simulink model "mbd_example_timer"  (R2022b)
settings: Solver=FixedStepDiscrete  StartTime=0.0  StopTime=10.0  RelTol=1e-3  EnableMultiTasking=on
PostLoadFcn:
  | run([bdroot '_init']);
InitFcn:
  | checkModelFolder(true); % Optional
  | run([bdroot '_init']);
values from neighbouring files (symbols this model uses):
  MBDDiag_Comm_Module = [2 3]    [mbd_example_timer_init.m]
  MBDDiag_Comm_Speed = [921600 921600]    [mbd_example_timer_init.m]
  MBDDiag_Comm_Type = [1 1]    [mbd_example_timer_init.m]
  T_s_LED1 = 1/LED1_Hz    (= 0.5)    [mbd_example_timer_init.m]
  T_s_LED2 = 1/LED2_Hz    (= 1)    [mbd_example_timer_init.m]
libraries: MbdLib_Uart x10, MbdLib_Timer x8, MbdLib_Digital x6, MbdLib_PortalDiag x4, MbdLib_SnapDiag x2, MbdLib_Required x1
settings Model: Creator=KenYoshioka  LastModifiedBy=KenYoshioka
settings SolverCC: AutoInsertRateTranBlk=on
settings OptimizationCC: DefaultParameterBehavior=Inlined  DefaultUnderspecifiedDataType=single  EnhancedBackFolding=on  BooleansAsBitfields=on  PassReuseOutputArgsAs=Individual arguments  ZeroExternalMemoryAtStartup=off  ZeroInternalMemoryAtStartup=off  OptimizeBlockOrder=speed  DifferentSizesBufferReuse=on  EfficientTunableParamExpr=on
settings DebuggingCC: ParameterTunabilityLossMsg=error
settings HardwareCC: ProdBitPerPointer=32  ProdBitPerSizeT=32  ProdBitPerPtrDiffT=32  ProdLargestAtomicInteger=Long  ProdLargestAtomicFloat=Double  ProdWordSize=32  ProdHWDeviceType=ARM Compatible->ARM Cortex-M
settings ModelReferenceCC: ModelReferenceNumInstancesAllowed=Single
settings SFSimCC: MATLABDynamicMemAlloc=off
settings RTWCC: Description=MBD Embedded Target STM32 Cortex M4 (real-time)  SystemTargetFile=MBD_STM32_stf.tlc  TemplateMakefile=MBD_STM32.tmf  Toolchain=arm-none-eabi - v10.3
settings CodeAppCC: ForceParamTrailComments=on  IgnoreCustomStorageClasses=off  MaxIdLength=255  OperatorAnnotations=on  SimulinkDataObjDesc=on  SFDataObjDesc=on  InsertBlockDesc=on
settings STFCustomTargetCC: MultiwordLength=256  IncludeMdlTerminateFcn=off  CombineOutputUpdateFcns=on  CombineSignalStateStructs=on  SuppressErrorStatus=on  ERTCustomFileBanners=on  SupportContinuousTime=off  RemoveResetFunc=on  MATLABClassNameForMDSCustomization=Simulink.SoftwareTarget.ERTCustomization  UseToolchainInfoCompliant=on  SystemTargetFile=MBD_STM32_stf.tlc
settings ERTTargetCC: ParMdlRefBuildCompliant=off  CompOptLevelCompliant=off  ConcurrentExecutionCompliant=off  IncludeMdlTerminateFcn=off  CombineSignalStateStructs=on  SuppressErrorStatus=on  SupportNonInlinedSFcns=on  ModelStepFunctionPrototypeControlCompliant=off  CPPClassGenCompliant=off  ExtModeStaticAllocSize=2000  InlinedParameterPlacement=NonHierarchical  ERTCustomFileTemplate=mbd_lib_interface.tlc  MaxLineWidth=110

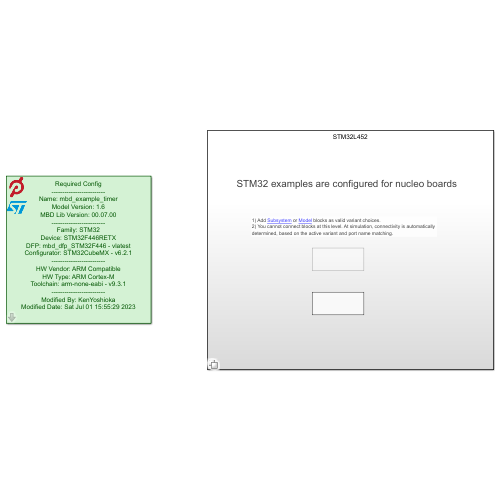
[thumbnail: Simulink's stored preview of the top-level diagram]
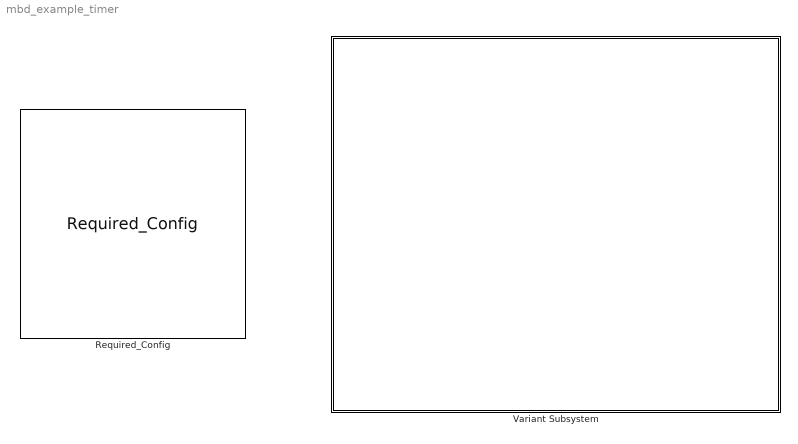
== system mbd_example_timer ==
  Required_Config : MbdLib_Required/Required_Config  Tag=MBD_Target_Info  Param_update=1
      settings: SourceProductName=Peloton Interface Library
  Variant Subsystem : Subsystem  Variant=on

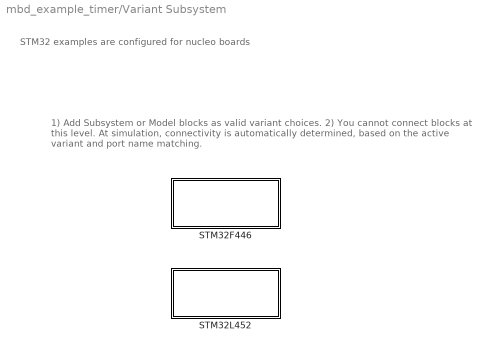
== system mbd_example_timer/Variant Subsystem ==
  note: STM32 examples are configured for nucleo boards
  note: 1) Add Subsystem or Model blocks as valid variant choices.
      | 2) You cannot connect blocks at this level. At simulation, connectivity is automatically
      | determined, based on the active variant and port name matching.
  STM32F446 : Subsystem  VariantControl=VAR_MBD_STM32F446
  STM32L452 : Subsystem  VariantControl=VAR_MBD_STM32L452

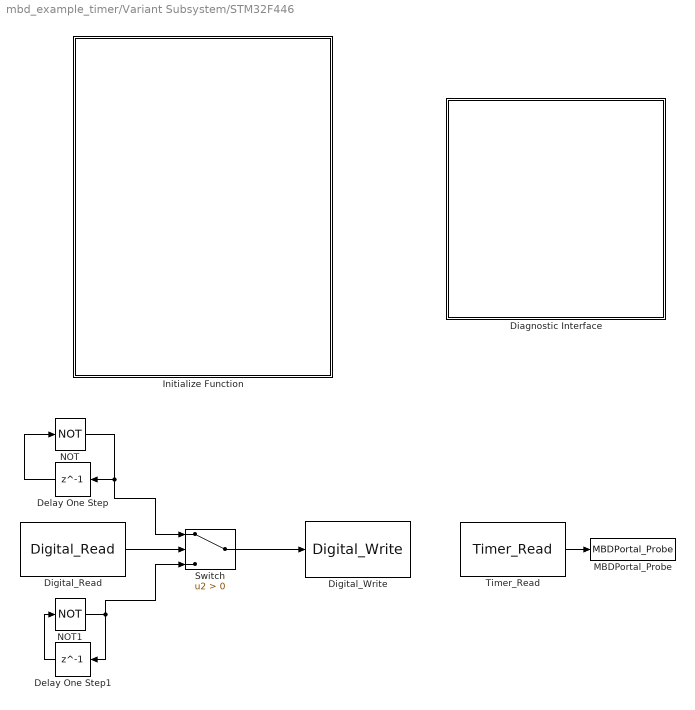
== system mbd_example_timer/Variant Subsystem/STM32F446 ==
  Delay One Step : Delay  DelayLength=1  SampleTime=T_s_LED1
  Delay One Step1 : Delay  DelayLength=1  SampleTime=T_s_LED2
  Diagnostic Interface : Subsystem
  Digital_Read : MbdLib_Digital/Digital_Read  Param_module=C  Param_ch=13  Param_sampleTime=-1  Sim_invert=off  Sim_out=0
      settings: SourceProductName=Peloton Interface Library
  Digital_Write : MbdLib_Digital/Digital_Write  Param_module=C  Param_ch=10  Param_sampleTime=-1
      settings: SourceProductName=Peloton Interface Library
  Initialize Function : Subsystem  TreatAsAtomicUnit=on
  MBDPortal_Probe : MbdLib_PortalDiag/MBDPortal_Probe  Param_SigNameInherited=on  Param_SigName=Timer_out  Param_SigIndex=0  Param_SigMax=MBDPortal_SignalNum  Param_SampleTime=MBDPortal_CommonSampleRate
      settings: SourceProductName=Peloton Component Library
  NOT : Logic  Operator=NOT  IconShape=distinctive  AllPortsSameDT=off  OutDataTypeStr=boolean
  NOT1 : Logic  Operator=NOT  IconShape=distinctive  AllPortsSameDT=off  OutDataTypeStr=boolean
  Switch : Switch  Criteria=u2 > Threshold  SaturateOnIntegerOverflow=off  InputSameDT=off
  Timer_Read : MbdLib_Timer/Timer_Read  Param_module=6  Param_ch=0  Param_sampleTime=-1
      settings: SourceProductName=Peloton Interface Library
  wires:
  NOT1/1 -> Switch/3, Delay One Step1/1
  NOT/1 -> Switch/1, Delay One Step/1
  Delay One Step/1 -> NOT/1
  Delay One Step1/1 -> NOT1/1
  Digital_Read/1 -> Switch/2
  Switch/1 -> Digital_Write/1
  Timer_Read/1 -> MBDPortal_Probe/1

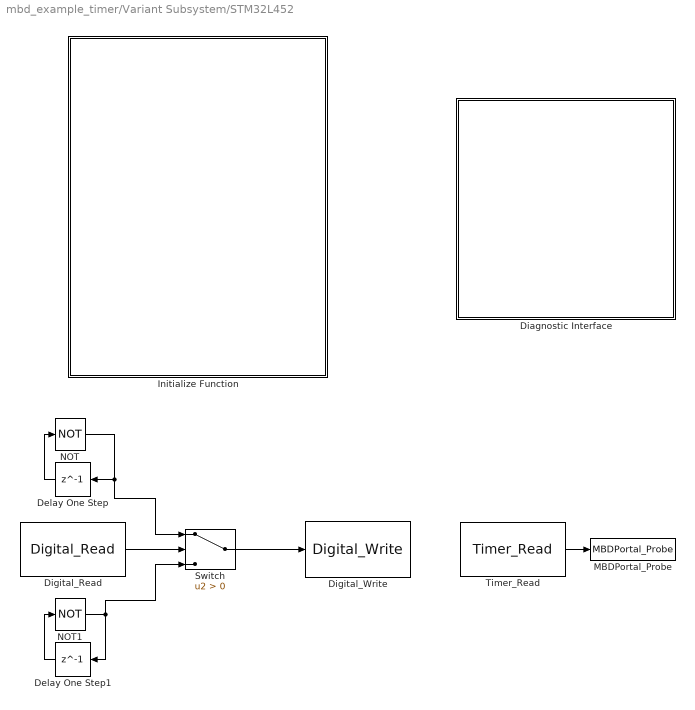
== system mbd_example_timer/Variant Subsystem/STM32L452 ==
  Delay One Step : Delay  DelayLength=1  SampleTime=T_s_LED1
  Delay One Step1 : Delay  DelayLength=1  SampleTime=T_s_LED2
  Diagnostic Interface : Subsystem
  Digital_Read : MbdLib_Digital/Digital_Read  Param_module=C  Param_ch=13  Param_sampleTime=-1  Sim_invert=off  Sim_out=0
      settings: SourceProductName=Peloton Interface Library
  Digital_Write : MbdLib_Digital/Digital_Write  Param_module=C  Param_ch=10  Param_sampleTime=-1
      settings: SourceProductName=Peloton Interface Library
  Initialize Function : Subsystem  TreatAsAtomicUnit=on
  MBDPortal_Probe : MbdLib_PortalDiag/MBDPortal_Probe  Param_SigNameInherited=on  Param_SigName=Timer_out  Param_SigIndex=0  Param_SigMax=MBDPortal_SignalNum  Param_SampleTime=MBDPortal_CommonSampleRate
      settings: SourceProductName=Peloton Component Library
  NOT : Logic  Operator=NOT  IconShape=distinctive  AllPortsSameDT=off  OutDataTypeStr=boolean
  NOT1 : Logic  Operator=NOT  IconShape=distinctive  AllPortsSameDT=off  OutDataTypeStr=boolean
  Switch : Switch  Criteria=u2 > Threshold  SaturateOnIntegerOverflow=off  InputSameDT=off
  Timer_Read : MbdLib_Timer/Timer_Read  Param_module=16  Param_ch=0  Param_sampleTime=-1
      settings: SourceProductName=Peloton Interface Library
  wires:
  NOT1/1 -> Switch/3, Delay One Step1/1
  NOT/1 -> Switch/1, Delay One Step/1
  Delay One Step/1 -> NOT/1
  Delay One Step1/1 -> NOT1/1
  Digital_Read/1 -> Switch/2
  Switch/1 -> Digital_Write/1
  Timer_Read/1 -> MBDPortal_Probe/1

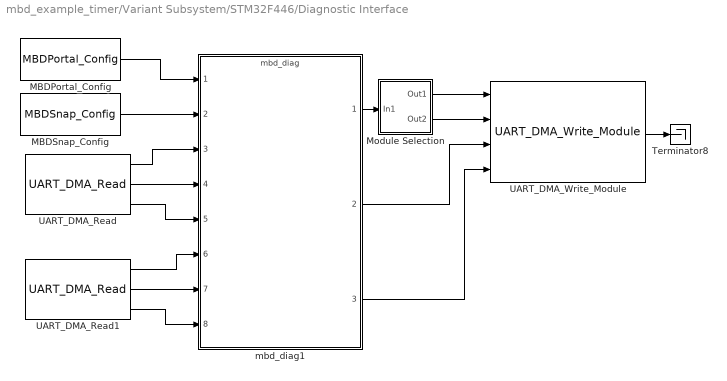
== system mbd_example_timer/Variant Subsystem/STM32F446/Diagnostic Interface ==
  MBDPortal_Config : MbdLib_PortalDiag/MBDPortal_Config  Param_SigMax=MBDPortal_SignalNum  Param_ParamMax=MBDPortal_ParamNum
      settings: SourceProductName=Peloton Component Library
  MBDSnap_Config : MbdLib_SnapDiag/MBDSnap_Config  Priority=-5000  Param_enableAll=on  Param_SampleTime=T_s_COMM  Param_SigMax=MBDSnap_SignalNum
      settings: SourceProductName=Peloton Component Library
  Module Selection : Subsystem
  Terminator8 : Terminator
  UART_DMA_Read : MbdLib_Uart/UART_DMA_Read  Tag=TAG_UART_DMA  Param_module=MBDDiag_Comm_Module(1)  Param_type=USART  Param_readLim=100  Param_sampleTime=T_s_COMM
      settings: SourceProductName=Peloton Interface Library
  UART_DMA_Read1 : MbdLib_Uart/UART_DMA_Read  Tag=TAG_UART_DMA  Param_module=MBDDiag_Comm_Module(2)  Param_type=USART  Param_readLim=100  Param_sampleTime=T_s_COMM
      settings: SourceProductName=Peloton Interface Library
  UART_DMA_Write_Module : MbdLib_Uart/UART_DMA_Write_Module  Param_instanceNum=2  Param_module1=MBDDiag_Comm_Module(1)  Param_type1=USART  Param_module2=MBDDiag_Comm_Module(2)  Param_type2=USART  Param_module3=0  Param_type3=UART  Param_module4=0  Param_type4=UART  Param_sampleTime=-1  Sim_status=0
      settings: SourceProductName=Peloton Interface Library
  mbd_diag1 : ModelReference  ModelNameDialog=mbd_diag.slx  SimulationMode=Normal  ModelReferenceVersion=2.294  SimulationMode=Normal
  wires:
  Module Selection/2(Out2) -> UART_DMA_Write_Module/2
  UART_DMA_Read1/2 -> mbd_diag1/7
  UART_DMA_Read/1 -> mbd_diag1/3
  UART_DMA_Write_Module/1 -> Terminator8/1
  mbd_diag1/1 -> Module Selection/1(In1)
  MBDPortal_Config/1 -> mbd_diag1/1
  mbd_diag1/3 -> UART_DMA_Write_Module/4
  MBDSnap_Config/1 -> mbd_diag1/2
  mbd_diag1/2 -> UART_DMA_Write_Module/3
  UART_DMA_Read/2 -> mbd_diag1/4
  Module Selection/1(Out1) -> UART_DMA_Write_Module/1
  UART_DMA_Read1/1 -> mbd_diag1/6
  UART_DMA_Read/3 -> mbd_diag1/5
  UART_DMA_Read1/3 -> mbd_diag1/8

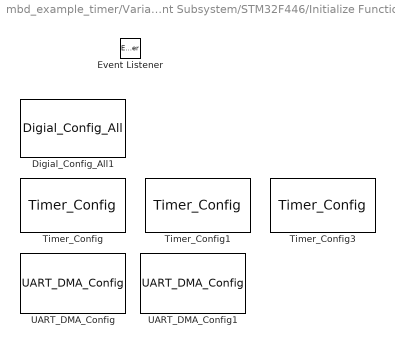
== system mbd_example_timer/Variant Subsystem/STM32F446/Initialize Function ==
  Digial_Config_All1 : MbdLib_Digital/Digial_Config_All  Priority=30  Param_channels={ 'A', '0', 'off', '0 : input', '0 : low', '0 : none', '0 : none', '0 : low', '0 : low'; 'A', '1', 'off', '0 : input', '0 : low', '0 : none', '0 : none', '0 : low', '0 : low'; 'A', '2', 'off', '0 : input', '0 : low', '0 : none', '0 : none', '0 : low', '0 : low'; 'A', '3', 'off', '0 : input', '0 : low', '0 : none', '0 : none', '0 : low', '0 : low'; 'A', '4', 'off', '0 : input', '0 : low', '0 : none', '0 : none', '0 : low', '0 : low'; 'A', '5', 'off', '0 : input', '0 : low', '0 : none', '0 : none', '0 : low', '0 : low'; 'A', '6', 'off', '0 : input', '0 : low', '0 : none', '0 : none', '0 : low', '0 : low'; 'A', '7', 'off', '0 : input', '0 : low', '0 : none', '0 : none', '0 : low', '0 : low'; 'A', '8', 'off', '0 : input', '0 : low', '0 : none', '0 : none', '0 : low', '0 : low'; 'A', '9', 'off', '0 : input', '0 : low', '0 : none', '0 : none', '0 : low', '0 : low'; 'A', '10', 'off', '0 : input', '0 : low', '0 : none', '0 : none', '0 : low', '0 : low'; 'A', '11', 'off', '0 : input', '0 : low', '0 : none', '0 : none', '0 : low', '0 : low'; 'A', '12', 'off', '0 : input', '0 : low', '0 : none', '0 : none', '0 : low', '0 : low'; 'A', '13', 'off', '0 : input', '0 : low', '0 : none', '0 : none', '0 : low', '0 : low'; 'A', '14', 'off', '0 : input', '0 : low', '0 : none', '0 : none', '0 : low', '0 : low'; 'A', '15', 'off', '0 : input', '0 : low', '0 : none', '0 : none', '0 : low', '0 : low'; 'A', '16', 'off', '0 : input', '0 : low', '0 : none', '0 : none', '0 : low', '0 : low'; 'A', '17', 'off', '0 : input', '0 : low', '0 : none', '0 : none', '0 : low', '0 : low'; 'A', '18', 'off', '0 : input', '0 : low', '0 : none', '0 : none', '0 : low', '0 : low'; 'A', '19', 'off', '0 : input', '0 : low', '0 : none', '0 : none', '0 : low', '0 : low'; 'A', '20', 'off', '0 : input', '0 : low', '0 : none', '0 : none', '0 : low', '0 : low'; 'A', '21', 'off', '0 : input', '0 : low', '0 : none', '0 : none', '0 : low', '0 : low'; 'A', '22', 'off', '0 : input', '0 : low', '0 : none', '0 : none', '0 : low', '0 : low'; 'A', '23', 'off', '0 : input', '0 : low', '0 : none', '0 : none', '0 : low', '0 : low'; 'A', '24', 'off', '0 : input', '0 : low', '0 : none', '0 : none', '0 : low', '0 : low'; 'A', '25', 'off', '0 : input', '0 : low', '0 : none', '0 : none', '0 : low', '0 : low'; 'A', '26', 'off', '0 : input', '0 : low', '0 : none', '0 : none', '0 : low', '0 : low'; 'A', '27', 'off', '0 : input', '0 : low', '0 : none', '0 : none', '0 : low', '0 : low'; 'A', '28', 'off', '0 : input', '0 : low', '0 : none', '0 : none', '0 : low', '0 : low'; 'A', '29', 'off', '0 : input', '0 : low', '0 : none', '0 : none', '0 : low', '0 : low'; 'A', '30', 'off', '0 : input', '0 : low', '0 : none', '0 : none', '0 : low', '0 : low'; 'A', '31', 'off', '0 : input', '0 : low', '0 : none', '0 : none', '0 : low', '0 : low'; 'B', '0', 'off', '0 : input', '0 : low', '0 : none', '0 : none', '0 : low', '0 : low'; 'B', '1', 'off', '0 : input', '0 : low', '0 : none', '0 : none', '0 : low', '0 : low'; 'B', '2', 'off', '0 : input', '0 : low', '0 : none', '0 : none', '0 : low', '0 : low'; 'B', '3', 'off', '0 : input', '0 : low', '0 : none', '0 : none', '0 : low', '0 : low'; 'B', '4', 'off', '0 : input', '0 : low', '0 : none', '0 : none', '0 : low', '0 : low'; 'B', '5', 'off', '0 : input', '0 : low', '0 : none', '0 : none', '0 : low', '0 : low'; 'B', '6', 'off', '0 : input', '0 : low', '0 : none', '0 : none', '0 : low', '0 : low'; 'B', '7', 'off', '0 : input', '0 : low', '0 : none', '0 : none', '0 : low', '0 : low'; 'B', '8', 'off', '0 : input', '0 : low', '0 : none', '0 : none', '0 : low', '0 : low'; 'B', '9', 'off', '0 : input', '0 : low', '0 : none', '0 : none', '0 : low', '0 : low'; 'B', '10', 'off', '0 : input', '0 : low', '0 : none', '0 : none', '0 : low', '0 : low'; 'B', '11', 'off', '0 : input', '0 : low', '0 : none', '0 : none', '0 : low', '0 : low'; 'B', '12', 'off', '0 : input', '0 : low', '0 : none', '0 : none', '0 : low', '0 : low'; 'B', '13', 'off', '0 : input', '0 : low', '0 : none', '0 : none', '0 : low', '0 : low'; 'C', '0', 'off', '0 : input', '0 : low', '0 : none', '0 : none', '0 : low', '0 : low'; 'C', '1', 'off', '0 : input', '0 : low', '0 : none', '0 : none', '0 : low', '0 : low'; 'C', '2', 'off', '0 : input', '0 : low', '0 : none', '0 : none', '0 : low', '0 : low'; 'C', '3', 'off', '0 : input', '0 : low', '0 : none', '0 : none', '0 : low', '0 : low'; 'C', '4', 'off', '0 : input', '0 : low', '0 : none', '0 : none', '0 : low', '0 : low'; 'C', '5', 'off', '0 : input', '0 : low', '0 : none', '0 : none', '0 : low', '0 : low'; 'C', '6', 'off', '0 : input', '0 : low', '0 : none', '0 : none', '0 : low', '0 : low'; 'C', '7', 'off', '0 : input', '0 : low', '0 : none', '0 : none', '0 : low', '0 : low'; 'C', '8', 'off', '0 : input', '0 : low', '0 : none', '0 : none', '0 : low', '0 : low'; 'C', '9', 'off', '0 : input', '0 : low', '0 : none', '0 : none', '0 : low', '0 : low'; 'C', '10', 'on', '1 : output', '0 : low', '0 : none', '0 : none', '0 : low', '0 : low'; 'C', '11', 'off', '0 : input', '0 : low', '0 : none', '0 : none', '0 : low', '0 : low'; 'C', '12', 'off', '0 : input', '0 : low', '0 : none', '0 : none', '0 : low', '0 : low'; 'C', '13', 'on', '0 : input', '0 : low', '0 : none', '1 : pullup', '0 : low', '0 : low'; 'C', '14', 'off', '0 : input', '0 : low', '0 : none', '0 : none', '0 : low', '0 : low'; 'C', '15', 'off', '0 : input', '0 : low', '0 : none', '0 : none', '0 : low', '0 : low'; 'C', '16', 'off', '0 : input', '0 : low', '0 : none', '0 : none', '0 : low', '0 : low'; 'C', '17', 'off', '0 : input', '0 : low', '0 : none', '0 : none', '0 : low', '0 : low'; 'C', '18', 'off', '0 : input', '0 : low', '0 : none', '0 : none', '0 : low', '0 : low'; 'C', '19', 'off', '0 : input', '0 : low', '0 : none', '0 : none', '0 : low', '0 : low'; 'C', '20', 'off', '0 : input', '0 : low', '0 : none', '0 : none', '0 : low', '0 : low'; 'C', '21', 'off', '0 : input', '0 : low', '0 : none', '0 : none', '0 : low', '0 : low'; 'C', '22', 'off', '0 : input', '0 : low', '0 : none', '0 : none', '0 : low', '0 : low'; 'C', '23', 'off', '0 : input', '0 : low', '0 : none', '0 : none', '0 : low', '0 : low'; 'C', '24', 'off', '0 : input', '0 : low', '0 : none', '0 : none', '0 : low', '0 : low'; 'C', '25', 'off', '0 : input', '0 : low', '0 : none', '0 : none', '0 : low', '0 : low'; 'C', '26', 'off', '0 : input', '0 : low', '0 : none', '0 : none', '0 : low', '0 : low'; 'C', '27', 'off', '0 : input', '0 : low', '0 : none', '0 : none', '0 : low', '0 : low'; 'C', '28', 'off', '0 : input', '0 : low', '0 : none', '0 : none', '0 : low', '0 : low'; 'C', '29', 'off', '0 : input', '0 : low', '0 : none', '0 : none', '0 : low', '0 : low'; 'C', '30', 'off', '0 : input', '0 : low', '0 : none', '0 : none', '0 : low', '0 : low'; 'C', '31', 'off', '0 : input', '0 : low', '0 : none', '0 : none', '0 : low', '0 : low'; 'D', '0', 'off', '0 : input', '0 : low', '0 : none', '0 : none', '0 : low', '0 : low'; 'D', '1', 'off', '0 : input', '0 : low', '0 : none', '0 : none', '0 : low', '0 : low'; 'D', '2', 'off', '0 : input', '0 : low', '0 : none', '0 : none', '0 : low', '0 : low'; 'D', '3', 'off', '0 : input', '0 : low', '0 : none', '0 : none', '0 : low', '0 : low'; 'D', '4', 'off', '0 : input', '0 : low', '0 : none', '0 : none', '0 : low', '0 : low'; 'D', '5', 'off', '0 : input', '0 : low', '0 : none', '0 : none', '0 : low', '0 : low'; 'D', '6', 'off', '0 : input', '0 : low', '0 : none', '0 : none', '0 : low', '0 : low'; 'D', '7', 'off', '0 : input', '0 : low', '0 : none', '0 : none', '0 : low', '0 : low'; 'D', '8', 'off', '0 : input', '0 : low', '0 : none', '0 : none', '0 : low', '0 : low'; 'D', '9', 'off', '0 : input', '0 : low', '0 : none', '0 : none', '0 : low', '0 : low'; 'D', '10', 'off', '0 : input', '0 : low', '0 : none', '0 : none', '0 : low', '0 : low'; 'D', '11', 'off', '0 : input', '0 : low', '0 : none', '0 : none', '0 : low', '0 : low'; 'D', '12', 'off', '0 : input', '0 : low', '0 : none', '0 : none', '0 : low', '0 : low'; 'D', '13', 'off', '0 : input', '0 : low', '0 : none', '0 : none', '0 : low', '0 : low'; 'D', '14', 'off', '0 : input', '0 : low', '0 : none', '0 : none', '0 : low', '0 : low'; 'D', '15', 'off', '0 : input', '0 : low', '0 : none', '0 : none', '0 : low', '0 : low'; 'D', '16', 'off', '0 : input', '0 : low', '0 : none', '0 : none', '0 : low', '0 : low'; 'D', '17', 'off', '0 : input', '0 : low', '0 : none', '0 : none', '0 : low', '0 : low'; 'D', '18', 'off', '0 : input', '0 : low', '0 : none', '0 : none', '0 : low', '0 : low'; 'D', '19', 'off', '0 : input', '0 : low', '0 : none', '0 : none', '0 : low', '0 : low'; 'D', '20', 'off', '0 : input', '0 : low', '0 : none', '0 : none', '0 : low', '0 : low'; 'D', '21', 'off', '0 : input', '0 : low', '0 : none', '0 : none', '0 : low', '0 : low'; 'D', '22', 'off', '0 : input', '0 : low', '0 : none', '0 : none', '0 : low', '0 : low'; 'D', '23', 'off', '0 : input', '0 : low', '0 : none', '0 : none', '0 : low', '0 : low'; 'D', '24', 'off', '0 : input', '0 : low', '0 : none', '0 : none', '0 : low', '0 : low'; 'D', '25', 'off', '0 : input', '0 : low', '0 : none', '0 : none', '0 : low', '0 : low'; 'D', '26', 'off', '0 : input', '0 : low', '0 : none', '0 : none', '0 : low', '0 : low'; 'D', '27', 'off', '0 : input', '0 : low', '0 : none', '0 : none', '0 : low', '0 : low'; 'D', '28', 'off', '0 : input', '0 : low', '0 : none', '0 : none', '0 : low', '0 : low'; 'D', '29', 'off', '0 : input', '0 : low', '0 : none', '0 : none', '0 : low', '0 : low'; 'D', '30', 'off', '0 : input', '0 : low', '0 : none', '0 : none', '0 : low', '0 : low'; 'D', '31', 'off', '0 : input', '0 : low', '0 : none', '0 : none', '0 : low', '0 : low'; 'E', '0', 'off', '0 : input', '0 : low', '0 : none', '0 : none', '0 : low', '0 : low'; 'E', '1', 'off', '0 : input', '0 : low', '0 : none', '0 : none', '0 : low', '0 : low'; 'E', '2', 'off', '0 : input', '0 : low', '0 : none', '0 : none', '0 : low', '0 : low'; 'E', '3', 'off', '0 : input', '0 : low', '0 : none', '0 : none', '0 : low', '0 : low'; 'E', '4', 'off', '0 : input', '0 : low', '0 : none', '0 : none', '0 : low', '0 : low'; 'E', '5', 'off', '0 : input', '0 : low', '0 : none', '0 : none', '0 : low', '0 : low' }  Param_priority=30  Param_sampleTime=-1
      settings: AttributesFormatString=priority=%<priority>  SourceProductName=Peloton Interface Library
  Event Listener : EventListener  DisableCoverage=on  EventName=reset
  Timer_Config : MbdLib_Timer/Timer_Config  Priority=100  Param_update=1  Param_module=1  Param_step=0  Param_period=Comm_period_cycles  Param_divider=Comm_clock_divider  Param_step0=0  Param_clksrc0=0  Param_period0=LED1_period_cycles  Param_divider0=LED1_clock_divider  Param_step1=-1  Param_clksrc1=0  Param_period1=0  Param_divider1=0  Param_step2=-1  Param_clksrc2=0  Param_period2=0  Param_divider2=0  Param_priority=100  Param_sampleTime=-1
      settings: AttributesFormatString=priority=%<priority>  SourceProductName=Peloton Interface Library
  Timer_Config1 : MbdLib_Timer/Timer_Config  Priority=101  Param_update=1  Param_module=6  Param_step=1  Param_period=LED1_period_cycles  Param_divider=LED1_clock_divider  Param_step0=1  Param_clksrc0=0  Param_period0=LED2_period_cycles  Param_divider0=LED2_clock_divider  Param_step1=-1  Param_clksrc1=0  Param_period1=0  Param_divider1=0  Param_step2=-1  Param_clksrc2=0  Param_period2=0  Param_divider2=0  Param_priority=101  Param_sampleTime=-1
      settings: AttributesFormatString=priority=%<priority>  SourceProductName=Peloton Interface Library
  Timer_Config3 : MbdLib_Timer/Timer_Config  Priority=102  Param_update=1  Param_module=7  Param_step=2  Param_period=LED2_period_cycles  Param_divider=LED2_clock_divider  Param_step0=2  Param_clksrc0=0  Param_period0=LED2_period_cycles  Param_divider0=LED2_clock_divider  Param_step1=-1  Param_clksrc1=0  Param_period1=0  Param_divider1=0  Param_step2=-1  Param_clksrc2=0  Param_period2=0  Param_divider2=0  Param_priority=102  Param_sampleTime=-1
      settings: AttributesFormatString=priority=%<priority>  SourceProductName=Peloton Interface Library
  UART_DMA_Config : MbdLib_Uart/UART_DMA_Config  Priority=110  Param_module=MBDDiag_Comm_Module(1)  Param_type=USART  Param_speed=MBDDiag_Comm_Speed(1)  Param_dataBits=8  Param_stopBits=1  Param_parity=None  Param_priority=110  Param_sampleTime=-1
      settings: AttributesFormatString=priority=%<priority>  SourceProductName=Peloton Interface Library
  UART_DMA_Config1 : MbdLib_Uart/UART_DMA_Config  Priority=110  Param_module=MBDDiag_Comm_Module(2)  Param_type=USART  Param_speed=MBDDiag_Comm_Speed(2)  Param_dataBits=8  Param_stopBits=1  Param_parity=None  Param_priority=110  Param_sampleTime=-1
      settings: AttributesFormatString=priority=%<priority>  SourceProductName=Peloton Interface Library

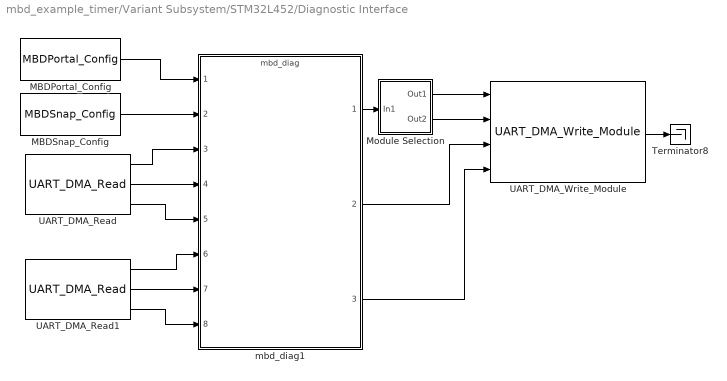
== system mbd_example_timer/Variant Subsystem/STM32L452/Diagnostic Interface ==
  MBDPortal_Config : MbdLib_PortalDiag/MBDPortal_Config  Param_SigMax=MBDPortal_SignalNum  Param_ParamMax=MBDPortal_ParamNum
      settings: SourceProductName=Peloton Component Library
  MBDSnap_Config : MbdLib_SnapDiag/MBDSnap_Config  Priority=-5000  Param_enableAll=on  Param_SampleTime=T_s_COMM  Param_SigMax=MBDSnap_SignalNum
      settings: SourceProductName=Peloton Component Library
  Module Selection : Subsystem
  Terminator8 : Terminator
  UART_DMA_Read : MbdLib_Uart/UART_DMA_Read  Tag=TAG_UART_DMA  Param_module=MBDDiag_Comm_Module(1)  Param_type=USART  Param_readLim=100  Param_sampleTime=T_s_COMM
      settings: SourceProductName=Peloton Interface Library
  UART_DMA_Read1 : MbdLib_Uart/UART_DMA_Read  Tag=TAG_UART_DMA  Param_module=MBDDiag_Comm_Module(2)  Param_type=USART  Param_readLim=100  Param_sampleTime=T_s_COMM
      settings: SourceProductName=Peloton Interface Library
  UART_DMA_Write_Module : MbdLib_Uart/UART_DMA_Write_Module  Param_instanceNum=2  Param_module1=MBDDiag_Comm_Module(1)  Param_type1=USART  Param_module2=MBDDiag_Comm_Module(2)  Param_type2=USART  Param_module3=0  Param_type3=UART  Param_module4=0  Param_type4=UART  Param_sampleTime=-1  Sim_status=0
      settings: SourceProductName=Peloton Interface Library
  mbd_diag1 : ModelReference  ModelNameDialog=mbd_diag.slx  SimulationMode=Normal  ModelReferenceVersion=2.294  SimulationMode=Normal
  wires:
  Module Selection/2(Out2) -> UART_DMA_Write_Module/2
  UART_DMA_Read1/2 -> mbd_diag1/7
  UART_DMA_Read/1 -> mbd_diag1/3
  UART_DMA_Write_Module/1 -> Terminator8/1
  mbd_diag1/1 -> Module Selection/1(In1)
  MBDPortal_Config/1 -> mbd_diag1/1
  mbd_diag1/3 -> UART_DMA_Write_Module/4
  MBDSnap_Config/1 -> mbd_diag1/2
  mbd_diag1/2 -> UART_DMA_Write_Module/3
  UART_DMA_Read/2 -> mbd_diag1/4
  Module Selection/1(Out1) -> UART_DMA_Write_Module/1
  UART_DMA_Read1/1 -> mbd_diag1/6
  UART_DMA_Read/3 -> mbd_diag1/5
  UART_DMA_Read1/3 -> mbd_diag1/8

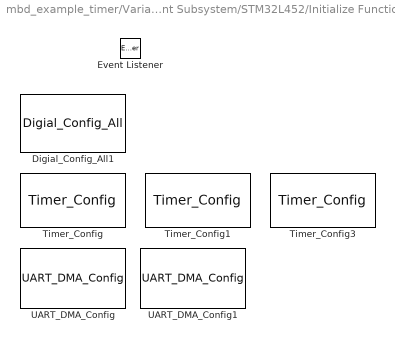
== system mbd_example_timer/Variant Subsystem/STM32L452/Initialize Function ==
  Digial_Config_All1 : MbdLib_Digital/Digial_Config_All  Priority=30  Param_channels={ 'A', '0', 'off', '0 : input', '0 : low', '0 : none', '0 : none', '0 : low', '0 : low'; 'A', '1', 'off', '0 : input', '0 : low', '0 : none', '0 : none', '0 : low', '0 : low'; 'A', '2', 'off', '0 : input', '0 : low', '0 : none', '0 : none', '0 : low', '0 : low'; 'A', '3', 'off', '0 : input', '0 : low', '0 : none', '0 : none', '0 : low', '0 : low'; 'A', '4', 'off', '0 : input', '0 : low', '0 : none', '0 : none', '0 : low', '0 : low'; 'A', '5', 'off', '0 : input', '0 : low', '0 : none', '0 : none', '0 : low', '0 : low'; 'A', '6', 'off', '0 : input', '0 : low', '0 : none', '0 : none', '0 : low', '0 : low'; 'A', '7', 'off', '0 : input', '0 : low', '0 : none', '0 : none', '0 : low', '0 : low'; 'A', '8', 'off', '0 : input', '0 : low', '0 : none', '0 : none', '0 : low', '0 : low'; 'A', '9', 'off', '0 : input', '0 : low', '0 : none', '0 : none', '0 : low', '0 : low'; 'A', '10', 'off', '0 : input', '0 : low', '0 : none', '0 : none', '0 : low', '0 : low'; 'A', '11', 'off', '0 : input', '0 : low', '0 : none', '0 : none', '0 : low', '0 : low'; 'A', '12', 'off', '0 : input', '0 : low', '0 : none', '0 : none', '0 : low', '0 : low'; 'A', '13', 'off', '0 : input', '0 : low', '0 : none', '0 : none', '0 : low', '0 : low'; 'A', '14', 'off', '0 : input', '0 : low', '0 : none', '0 : none', '0 : low', '0 : low'; 'A', '15', 'off', '0 : input', '0 : low', '0 : none', '0 : none', '0 : low', '0 : low'; 'A', '16', 'off', '0 : input', '0 : low', '0 : none', '0 : none', '0 : low', '0 : low'; 'A', '17', 'off', '0 : input', '0 : low', '0 : none', '0 : none', '0 : low', '0 : low'; 'A', '18', 'off', '0 : input', '0 : low', '0 : none', '0 : none', '0 : low', '0 : low'; 'A', '19', 'off', '0 : input', '0 : low', '0 : none', '0 : none', '0 : low', '0 : low'; 'A', '20', 'off', '0 : input', '0 : low', '0 : none', '0 : none', '0 : low', '0 : low'; 'A', '21', 'off', '0 : input', '0 : low', '0 : none', '0 : none', '0 : low', '0 : low'; 'A', '22', 'off', '0 : input', '0 : low', '0 : none', '0 : none', '0 : low', '0 : low'; 'A', '23', 'off', '0 : input', '0 : low', '0 : none', '0 : none', '0 : low', '0 : low'; 'A', '24', 'off', '0 : input', '0 : low', '0 : none', '0 : none', '0 : low', '0 : low'; 'A', '25', 'off', '0 : input', '0 : low', '0 : none', '0 : none', '0 : low', '0 : low'; 'A', '26', 'off', '0 : input', '0 : low', '0 : none', '0 : none', '0 : low', '0 : low'; 'A', '27', 'off', '0 : input', '0 : low', '0 : none', '0 : none', '0 : low', '0 : low'; 'A', '28', 'off', '0 : input', '0 : low', '0 : none', '0 : none', '0 : low', '0 : low'; 'A', '29', 'off', '0 : input', '0 : low', '0 : none', '0 : none', '0 : low', '0 : low'; 'A', '30', 'off', '0 : input', '0 : low', '0 : none', '0 : none', '0 : low', '0 : low'; 'A', '31', 'off', '0 : input', '0 : low', '0 : none', '0 : none', '0 : low', '0 : low'; 'B', '0', 'off', '0 : input', '0 : low', '0 : none', '0 : none', '0 : low', '0 : low'; 'B', '1', 'off', '0 : input', '0 : low', '0 : none', '0 : none', '0 : low', '0 : low'; 'B', '2', 'off', '0 : input', '0 : low', '0 : none', '0 : none', '0 : low', '0 : low'; 'B', '3', 'off', '0 : input', '0 : low', '0 : none', '0 : none', '0 : low', '0 : low'; 'B', '4', 'off', '0 : input', '0 : low', '0 : none', '0 : none', '0 : low', '0 : low'; 'B', '5', 'off', '0 : input', '0 : low', '0 : none', '0 : none', '0 : low', '0 : low'; 'B', '6', 'off', '0 : input', '0 : low', '0 : none', '0 : none', '0 : low', '0 : low'; 'B', '7', 'off', '0 : input', '0 : low', '0 : none', '0 : none', '0 : low', '0 : low'; 'B', '8', 'off', '0 : input', '0 : low', '0 : none', '0 : none', '0 : low', '0 : low'; 'B', '9', 'off', '0 : input', '0 : low', '0 : none', '0 : none', '0 : low', '0 : low'; 'B', '10', 'off', '0 : input', '0 : low', '0 : none', '0 : none', '0 : low', '0 : low'; 'B', '11', 'off', '0 : input', '0 : low', '0 : none', '0 : none', '0 : low', '0 : low'; 'B', '12', 'off', '0 : input', '0 : low', '0 : none', '0 : none', '0 : low', '0 : low'; 'B', '13', 'off', '0 : input', '0 : low', '0 : none', '0 : none', '0 : low', '0 : low'; 'C', '0', 'off', '0 : input', '0 : low', '0 : none', '0 : none', '0 : low', '0 : low'; 'C', '1', 'off', '0 : input', '0 : low', '0 : none', '0 : none', '0 : low', '0 : low'; 'C', '2', 'off', '0 : input', '0 : low', '0 : none', '0 : none', '0 : low', '0 : low'; 'C', '3', 'off', '0 : input', '0 : low', '0 : none', '0 : none', '0 : low', '0 : low'; 'C', '4', 'off', '0 : input', '0 : low', '0 : none', '0 : none', '0 : low', '0 : low'; 'C', '5', 'off', '0 : input', '0 : low', '0 : none', '0 : none', '0 : low', '0 : low'; 'C', '6', 'off', '0 : input', '0 : low', '0 : none', '0 : none', '0 : low', '0 : low'; 'C', '7', 'off', '0 : input', '0 : low', '0 : none', '0 : none', '0 : low', '0 : low'; 'C', '8', 'off', '0 : input', '0 : low', '0 : none', '0 : none', '0 : low', '0 : low'; 'C', '9', 'off', '0 : input', '0 : low', '0 : none', '0 : none', '0 : low', '0 : low'; 'C', '10', 'on', '1 : output', '0 : low', '0 : none', '0 : none', '0 : low', '0 : low'; 'C', '11', 'off', '0 : input', '0 : low', '0 : none', '0 : none', '0 : low', '0 : low'; 'C', '12', 'off', '0 : input', '0 : low', '0 : none', '0 : none', '0 : low', '0 : low'; 'C', '13', 'on', '0 : input', '0 : low', '0 : none', '1 : pullup', '0 : low', '0 : low'; 'C', '14', 'off', '0 : input', '0 : low', '0 : none', '0 : none', '0 : low', '0 : low'; 'C', '15', 'off', '0 : input', '0 : low', '0 : none', '0 : none', '0 : low', '0 : low'; 'C', '16', 'off', '0 : input', '0 : low', '0 : none', '0 : none', '0 : low', '0 : low'; 'C', '17', 'off', '0 : input', '0 : low', '0 : none', '0 : none', '0 : low', '0 : low'; 'C', '18', 'off', '0 : input', '0 : low', '0 : none', '0 : none', '0 : low', '0 : low'; 'C', '19', 'off', '0 : input', '0 : low', '0 : none', '0 : none', '0 : low', '0 : low'; 'C', '20', 'off', '0 : input', '0 : low', '0 : none', '0 : none', '0 : low', '0 : low'; 'C', '21', 'off', '0 : input', '0 : low', '0 : none', '0 : none', '0 : low', '0 : low'; 'C', '22', 'off', '0 : input', '0 : low', '0 : none', '0 : none', '0 : low', '0 : low'; 'C', '23', 'off', '0 : input', '0 : low', '0 : none', '0 : none', '0 : low', '0 : low'; 'C', '24', 'off', '0 : input', '0 : low', '0 : none', '0 : none', '0 : low', '0 : low'; 'C', '25', 'off', '0 : input', '0 : low', '0 : none', '0 : none', '0 : low', '0 : low'; 'C', '26', 'off', '0 : input', '0 : low', '0 : none', '0 : none', '0 : low', '0 : low'; 'C', '27', 'off', '0 : input', '0 : low', '0 : none', '0 : none', '0 : low', '0 : low'; 'C', '28', 'off', '0 : input', '0 : low', '0 : none', '0 : none', '0 : low', '0 : low'; 'C', '29', 'off', '0 : input', '0 : low', '0 : none', '0 : none', '0 : low', '0 : low'; 'C', '30', 'off', '0 : input', '0 : low', '0 : none', '0 : none', '0 : low', '0 : low'; 'C', '31', 'off', '0 : input', '0 : low', '0 : none', '0 : none', '0 : low', '0 : low'; 'D', '0', 'off', '0 : input', '0 : low', '0 : none', '0 : none', '0 : low', '0 : low'; 'D', '1', 'off', '0 : input', '0 : low', '0 : none', '0 : none', '0 : low', '0 : low'; 'D', '2', 'off', '0 : input', '0 : low', '0 : none', '0 : none', '0 : low', '0 : low'; 'D', '3', 'off', '0 : input', '0 : low', '0 : none', '0 : none', '0 : low', '0 : low'; 'D', '4', 'off', '0 : input', '0 : low', '0 : none', '0 : none', '0 : low', '0 : low'; 'D', '5', 'off', '0 : input', '0 : low', '0 : none', '0 : none', '0 : low', '0 : low'; 'D', '6', 'off', '0 : input', '0 : low', '0 : none', '0 : none', '0 : low', '0 : low'; 'D', '7', 'off', '0 : input', '0 : low', '0 : none', '0 : none', '0 : low', '0 : low'; 'D', '8', 'off', '0 : input', '0 : low', '0 : none', '0 : none', '0 : low', '0 : low'; 'D', '9', 'off', '0 : input', '0 : low', '0 : none', '0 : none', '0 : low', '0 : low'; 'D', '10', 'off', '0 : input', '0 : low', '0 : none', '0 : none', '0 : low', '0 : low'; 'D', '11', 'off', '0 : input', '0 : low', '0 : none', '0 : none', '0 : low', '0 : low'; 'D', '12', 'off', '0 : input', '0 : low', '0 : none', '0 : none', '0 : low', '0 : low'; 'D', '13', 'off', '0 : input', '0 : low', '0 : none', '0 : none', '0 : low', '0 : low'; 'D', '14', 'off', '0 : input', '0 : low', '0 : none', '0 : none', '0 : low', '0 : low'; 'D', '15', 'off', '0 : input', '0 : low', '0 : none', '0 : none', '0 : low', '0 : low'; 'D', '16', 'off', '0 : input', '0 : low', '0 : none', '0 : none', '0 : low', '0 : low'; 'D', '17', 'off', '0 : input', '0 : low', '0 : none', '0 : none', '0 : low', '0 : low'; 'D', '18', 'off', '0 : input', '0 : low', '0 : none', '0 : none', '0 : low', '0 : low'; 'D', '19', 'off', '0 : input', '0 : low', '0 : none', '0 : none', '0 : low', '0 : low'; 'D', '20', 'off', '0 : input', '0 : low', '0 : none', '0 : none', '0 : low', '0 : low'; 'D', '21', 'off', '0 : input', '0 : low', '0 : none', '0 : none', '0 : low', '0 : low'; 'D', '22', 'off', '0 : input', '0 : low', '0 : none', '0 : none', '0 : low', '0 : low'; 'D', '23', 'off', '0 : input', '0 : low', '0 : none', '0 : none', '0 : low', '0 : low'; 'D', '24', 'off', '0 : input', '0 : low', '0 : none', '0 : none', '0 : low', '0 : low'; 'D', '25', 'off', '0 : input', '0 : low', '0 : none', '0 : none', '0 : low', '0 : low'; 'D', '26', 'off', '0 : input', '0 : low', '0 : none', '0 : none', '0 : low', '0 : low'; 'D', '27', 'off', '0 : input', '0 : low', '0 : none', '0 : none', '0 : low', '0 : low'; 'D', '28', 'off', '0 : input', '0 : low', '0 : none', '0 : none', '0 : low', '0 : low'; 'D', '29', 'off', '0 : input', '0 : low', '0 : none', '0 : none', '0 : low', '0 : low'; 'D', '30', 'off', '0 : input', '0 : low', '0 : none', '0 : none', '0 : low', '0 : low'; 'D', '31', 'off', '0 : input', '0 : low', '0 : none', '0 : none', '0 : low', '0 : low'; 'E', '0', 'off', '0 : input', '0 : low', '0 : none', '0 : none', '0 : low', '0 : low'; 'E', '1', 'off', '0 : input', '0 : low', '0 : none', '0 : none', '0 : low', '0 : low'; 'E', '2', 'off', '0 : input', '0 : low', '0 : none', '0 : none', '0 : low', '0 : low'; 'E', '3', 'off', '0 : input', '0 : low', '0 : none', '0 : none', '0 : low', '0 : low'; 'E', '4', 'off', '0 : input', '0 : low', '0 : none', '0 : none', '0 : low', '0 : low'; 'E', '5', 'off', '0 : input', '0 : low', '0 : none', '0 : none', '0 : low', '0 : low' }  Param_priority=30  Param_sampleTime=-1
      settings: AttributesFormatString=priority=%<priority>  SourceProductName=Peloton Interface Library
  Event Listener : EventListener  DisableCoverage=on  EventName=reset
  Timer_Config : MbdLib_Timer/Timer_Config  Priority=100  Param_update=1  Param_module=6  Param_step=0  Param_period=Comm_period_cycles  Param_divider=Comm_clock_divider  Param_step0=0  Param_clksrc0=0  Param_period0=LED1_period_cycles  Param_divider0=LED1_clock_divider  Param_step1=-1  Param_clksrc1=0  Param_period1=0  Param_divider1=0  Param_step2=-1  Param_clksrc2=0  Param_period2=0  Param_divider2=0  Param_priority=100  Param_sampleTime=-1
      settings: AttributesFormatString=priority=%<priority>  SourceProductName=Peloton Interface Library
  Timer_Config1 : MbdLib_Timer/Timer_Config  Priority=101  Param_update=1  Param_module=15  Param_step=1  Param_period=LED1_period_cycles  Param_divider=LED1_clock_divider  Param_step0=1  Param_clksrc0=0  Param_period0=LED2_period_cycles  Param_divider0=LED2_clock_divider  Param_step1=-1  Param_clksrc1=0  Param_period1=0  Param_divider1=0  Param_step2=-1  Param_clksrc2=0  Param_period2=0  Param_divider2=0  Param_priority=101  Param_sampleTime=-1
      settings: AttributesFormatString=priority=%<priority>  SourceProductName=Peloton Interface Library
  Timer_Config3 : MbdLib_Timer/Timer_Config  Priority=102  Param_update=1  Param_module=16  Param_step=2  Param_period=LED2_period_cycles  Param_divider=LED2_clock_divider  Param_step0=2  Param_clksrc0=0  Param_period0=LED2_period_cycles  Param_divider0=LED2_clock_divider  Param_step1=-1  Param_clksrc1=0  Param_period1=0  Param_divider1=0  Param_step2=-1  Param_clksrc2=0  Param_period2=0  Param_divider2=0  Param_priority=102  Param_sampleTime=-1
      settings: AttributesFormatString=priority=%<priority>  SourceProductName=Peloton Interface Library
  UART_DMA_Config : MbdLib_Uart/UART_DMA_Config  Priority=110  Param_module=MBDDiag_Comm_Module(1)  Param_type=USART  Param_speed=MBDDiag_Comm_Speed(1)  Param_dataBits=8  Param_stopBits=1  Param_parity=None  Param_priority=110  Param_sampleTime=-1
      settings: AttributesFormatString=priority=%<priority>  SourceProductName=Peloton Interface Library
  UART_DMA_Config1 : MbdLib_Uart/UART_DMA_Config  Priority=110  Param_module=MBDDiag_Comm_Module(2)  Param_type=USART  Param_speed=MBDDiag_Comm_Speed(2)  Param_dataBits=8  Param_stopBits=1  Param_parity=None  Param_priority=110  Param_sampleTime=-1
      settings: AttributesFormatString=priority=%<priority>  SourceProductName=Peloton Interface Library

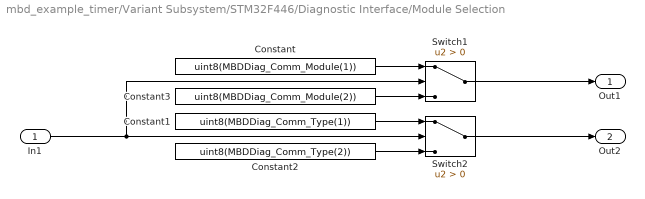
== system mbd_example_timer/Variant Subsystem/STM32F446/Diagnostic Interface/Module Selection ==
  In1 : Inport
  Constant : Constant  Value=uint8(MBDDiag_Comm_Module(1))
  Constant1 : Constant  Value=uint8(MBDDiag_Comm_Type(1))
  Constant2 : Constant  Value=uint8(MBDDiag_Comm_Type(2))
  Constant3 : Constant  Value=uint8(MBDDiag_Comm_Module(2))
  Switch1 : Switch  Criteria=u2 > Threshold  SaturateOnIntegerOverflow=off  InputSameDT=off
  Switch2 : Switch  Criteria=u2 > Threshold  SaturateOnIntegerOverflow=off  InputSameDT=off
  Out1 : Outport
  Out2 : Outport  Port=2
  wires:
  In1/1 -> Switch1/2, Switch2/2
  Constant3/1 -> Switch1/3
  Switch1/1 -> Out1/1
  Constant/1 -> Switch1/1
  Constant1/1 -> Switch2/1
  Switch2/1 -> Out2/1
  Constant2/1 -> Switch2/3

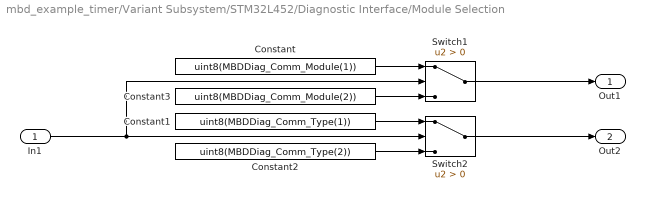
== system mbd_example_timer/Variant Subsystem/STM32L452/Diagnostic Interface/Module Selection ==
  In1 : Inport
  Constant : Constant  Value=uint8(MBDDiag_Comm_Module(1))
  Constant1 : Constant  Value=uint8(MBDDiag_Comm_Type(1))
  Constant2 : Constant  Value=uint8(MBDDiag_Comm_Type(2))
  Constant3 : Constant  Value=uint8(MBDDiag_Comm_Module(2))
  Switch1 : Switch  Criteria=u2 > Threshold  SaturateOnIntegerOverflow=off  InputSameDT=off
  Switch2 : Switch  Criteria=u2 > Threshold  SaturateOnIntegerOverflow=off  InputSameDT=off
  Out1 : Outport
  Out2 : Outport  Port=2
  wires:
  In1/1 -> Switch1/2, Switch2/2
  Constant3/1 -> Switch1/3
  Switch1/1 -> Out1/1
  Constant/1 -> Switch1/1
  Constant1/1 -> Switch2/1
  Switch2/1 -> Out2/1
  Constant2/1 -> Switch2/3
